simulink model "detect_rising_edge__simulation"  (R2017a)
settings: Solver=FixedStepAuto  StartTime=0.0  StopTime=3  RelTol=1e-3
libraries: simulink x1
settings Model: Creator=mini  LastModifiedBy=mini
settings DebuggingCC: SingleTaskRateTransMsg=error

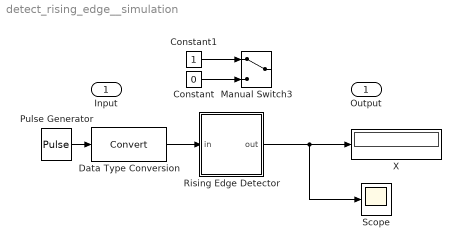
== system detect_rising_edge__simulation ==
  Input : Inport  OutDataTypeStr=boolean
  Constant : Constant  Value=0  OutDataTypeStr=boolean
  Constant1 : Constant  OutDataTypeStr=boolean
  Data Type Conversion : DataTypeConversion
  Manual Switch3 : ManualSwitch
  Pulse Generator : DiscretePulseGenerator  PulseType=Time based  Period=1  PulseWidth=50
  Rising Edge Detector : Subsystem
  Scope : Scope
  X : Display
  Output : Outport  OutDataTypeStr=boolean
  wires:
  Data Type Conversion/1 -> Rising Edge Detector/1(in)
  Rising Edge Detector/1(out) -> Scope/1, X/1
  Constant1/1 -> Manual Switch3/1
  Constant/1 -> Manual Switch3/2
  Pulse Generator/1 -> Data Type Conversion/1

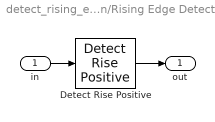
== system detect_rising_edge__simulation/Rising Edge Detector ==
  in : Inport  OutDataTypeStr=boolean
  Detect Rise Positive : simulink/Logic and Bit Operations/Detect Rise Positive  vinit=0  OutDataTypeStr=boolean
  out : Outport  OutDataTypeStr=boolean
  wires:
  in/1 -> Detect Rise Positive/1
  Detect Rise Positive/1 -> out/1
